simulink model "newModel"  (R2015b)
settings: Solver=VariableStepAuto  StartTime=0.0  StopTime=10  RelTol=1e-3
settings Model: Creator=Asus  LastModifiedBy=Asus

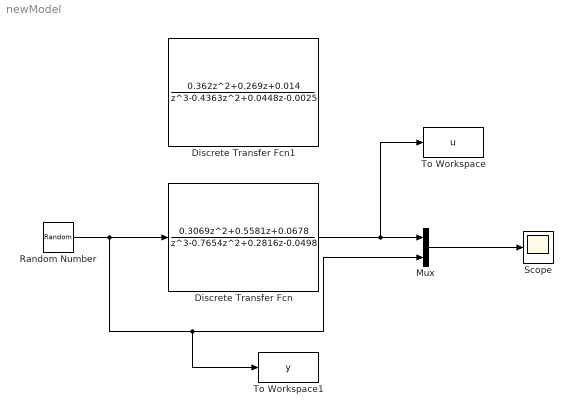
== system newModel ==
  Discrete Transfer Fcn : DiscreteTransferFcn  Numerator=[0 0.3069 0.5581 0.0678]  Denominator=[1 -0.7654 0.2816 -0.0498]
  Discrete Transfer Fcn1 : DiscreteTransferFcn  Numerator=[0 0.362 0.269 0.014]  Denominator=[1 -0.4363 0.0448 -0.0025]
  Mux : Mux  Inputs=2
  Random Number : RandomNumber  SampleTime=.1
  Scope : Scope
  To Workspace : ToWorkspace  VariableName=u  SampleTime=-1
  To Workspace1 : ToWorkspace  VariableName=y  SampleTime=-1
  wires:
  Random Number/1 -> Discrete Transfer Fcn/1, To Workspace1/1, Mux/2
  Discrete Transfer Fcn/1 -> To Workspace/1, Mux/1
  Mux/1 -> Scope/1
